simulink model "batterycharger_SOC"  (R2017b)
settings: Solver=VariableStepAuto  StartTime=0.0  StopTime=200  MaxStep=1e-4  RelTol=1e-3
undefined symbols (not defined in the file): Ion, Lithium
libraries: powerlib x8, electricdrivelib x2
settings Model: Creator=NGBNTA001  LastModifiedBy=NGBNTA001

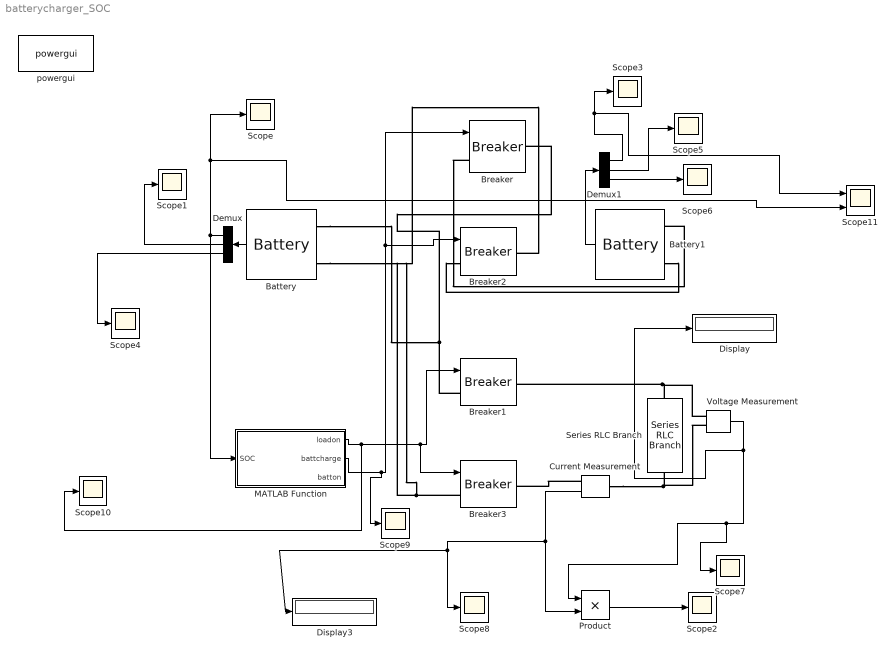
== system batterycharger_SOC ==
  Battery : electricdrivelib/Extra Sources/Battery  BatType=Lithium-Ion  ShowTempParam=off  ThermalPreset=no  ShowAgeParam=off  NomV=100  NomQ=5.4  SOC=88  Batt_Tr=30  PresetModel=on  MaxQ=5.4  MinV=75  FullV=116.3987  Dis_rate=2.3478  R=0.18519  Normal_OP=4.8835  expZone="[108.0386     0.2653043]"  current=[6.5 13 32.5]  Units=Time  Tci=20  NomT=20  T2=-30  MaxQ2=4.8  FullV2=7.1  Normal_OP2=5.655  expZone2="[6.58           1]"  Rca=0.6  ti=2000  Dp=0  Neq0=0  Tsim=1e6  Ta1=25  Qeol=5.4*0.9  Reol=0.013333*1.2  Char_age=[2.3478, 3]  Dis_age=[2.3478, 10]  N1=1500  N2=10500  N3=1000  N4=1400  Ta2=45  N5=950
  Battery1 : electricdrivelib/Extra Sources/Battery  BatType=Lithium-Ion  ShowTempParam=off  ThermalPreset=no  ShowAgeParam=off  NomV=100  NomQ=41.75  SOC=100  Batt_Tr=30  PresetModel=on  MaxQ=41.75  MinV=75  FullV=116.3987  Dis_rate=18.1522  R=0.023952  Normal_OP=37.7565  expZone="[108.0386      2.051196]"  current=[6.5 13 32.5]  Units=Time  Tci=20  NomT=20  T2=-30  MaxQ2=4.8  FullV2=7.1  Normal_OP2=5.655  expZone2="[6.58           1]"  Rca=0.6  ti=2000  Dp=0  Neq0=0  Tsim=1e6  Ta1=25  Qeol=5.4*0.9  Reol=0.013333*1.2  Char_age=[2.3478, 3]  Dis_age=[2.3478, 10]  N1=1500  N2=10500  N3=1000  N4=1400  Ta2=45  N5=950
  Breaker{,1..3} (4 alike) : powerlib/Elements/Breaker  InitialState=0  SwitchingTimes="[1/60  5/60]"  External=on  BreakerResistance=0.01  SnubberResistance=1e6  SnubberCapacitance=inf  Measurements=None  MoreParameters=on  NoBreakLoop=off
      settings: SourceProductName=Simscape Power Systems
  Current Measurement : powerlib/Measurements/Current Measurement  PhasorSimulation=off  OutputType=Complex  PSBequivalent=0
  Demux : Demux  Outputs=3
  Demux1 : Demux  Outputs=3
  Display : Display
  Display3 : Display
  MATLAB Function : MATLAB Function  TreatAsAtomicUnit=on
  Product : Product
  Scope{,1..10} (11 alike) : Scope
  Scope11 : Scope  NumInputPorts=2
  Series RLC Branch : powerlib/Elements/Series RLC Branch  LConnTagsString=__new0  RConnTagsString=__new0  BranchType=R  Resistance=5  Inductance=1e-3  SetiL0=off  InitialCurrent=0  Capacitance=1e-6  Setx0=off  InitialVoltage=0  Measurements=None
  Voltage Measurement : powerlib/Measurements/Voltage Measurement  PhasorSimulation=off  OutputType=Complex  PSBequivalent=0
  powergui : powerlib/powergui  Priority=1  SimulationMode=Continuous  SampleTime=50e-6  frequency=60  Iterations=50  frequencyindice=0  Pbase=100e6  ErrMax=1e-4  UnitsV=kV  UnitsW=MW  buscounter=0  FunctionMessages=off  echomessages=off  EnableUseOfTLC=off  CurrentSourceSwitches=off  DisableSnubberDevices=off  DisableRonSwitches=off  DisableVfSwitches=off  DisplayEquations=off  SolverType=Tustin/Backward Euler (TBE)  Interpol=off  ExternalGateDelay=off  methode=off  Ts=100  x0status=blocks  SPID=on  SwTol=0  HookPort=off  RestoreLinks=warning  ResistiveCurrentMeasurement=off  Frange=[0:2:500]  Ylog=off  Xlog=on  ShowGrid=off  save=off  variable=ZData  structure=0  ZoomFFT=off  StartTime=0.0  cycles=1  DisplayStyle=1  fundamental=60  FreqAxis=off  MaxFrequency=1000  frequencyindicesteady=1  RmsSteady=1  display=off
  wires:
  Current Measurement/1 -> Display3/1, Scope8/1, Product/2
  Voltage Measurement/1 -> Display/1, Scope7/1, Product/1
  MATLAB Function/2(battcharge) -> Scope9/1, Breaker2/1, Breaker/1
  MATLAB Function/1(loadon) -> Scope10/1, Breaker3/1, Breaker1/1
  Battery/1 -> Demux/1
  Demux/3 -> Scope4/1
  Demux/2 -> Scope1/1
  Demux/1 -> Scope11/2, Scope/1, MATLAB Function/1(SOC)
  Battery1/1 -> Demux1/1
  Demux1/1 -> Scope11/1, Scope3/1
  Demux1/2 -> Scope5/1
  Demux1/3 -> Scope6/1
  Product/1 -> Scope2/1
  connections:
  Series RLC Branch/LConn1 -- Voltage Measurement/LConn1 -- Breaker1/RConn1
  Current Measurement/RConn1 -- Breaker3/RConn1
  Current Measurement/LConn1 -- Voltage Measurement/LConn2 -- Series RLC Branch/RConn1
  Battery1/LConn2 -- Breaker2/LConn1
  Breaker3/LConn1 -- Battery/LConn2 -- Breaker2/RConn1
  Breaker/LConn1 -- Battery1/LConn1
  Breaker1/LConn1 -- Battery/LConn1 -- Breaker/RConn1

== matlab function batterycharger_SOC/MATLAB Function ==
  data: SOC input; loadon output; battcharge output; batton output
%This is the charge controller Algorithm for monitoring  the state of
%charge of the battery
function [loadon,battcharge,batton] = fcn(SOC)
loadon=1;
battcharge=0;
batton=0;
if (SOC>=235)  % if DC Voltage is greater than 235 V Disconnect battery
    loadon=1;  %  from PV-system
    batton=0;
    battcharge=1;
end
if (SOC<230) % if DC voltage is below 230V connect battery to PV-system
    loadon=1;
    batton=1;
    battcharge=0;
end
if (SOC>=20) % charge battery when the SOC is greater than 20 %
    loadon=1;
    battcharge=1;
end
if (SOC<20)   % disconnect (shutdown) battery if SOC is below 20%
    loadon=0;
    battcharge=1;
end
if (SOC>=90) %stop charging battery if SOC is greater than 90%
    loadon=1;
    battcharge=0;
end
